simulink model "robot_uniciclo"  (R2025a)
settings: Solver=VariableStepAuto  StartTime=0.0  StopTime=10.0  RelTol=1e-3
settings Model: Creator=Bremdow  LastModifiedBy=Bremdow

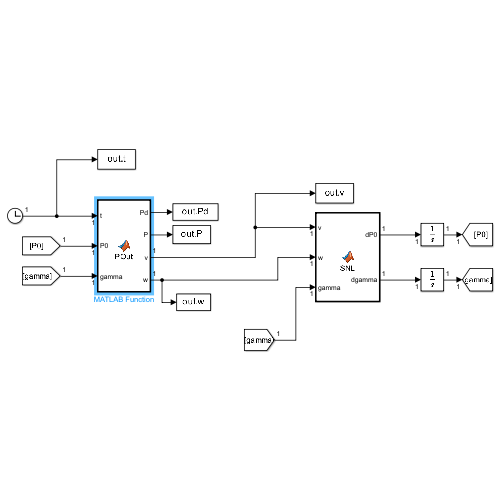
[thumbnail: Simulink's stored preview of the top-level diagram]
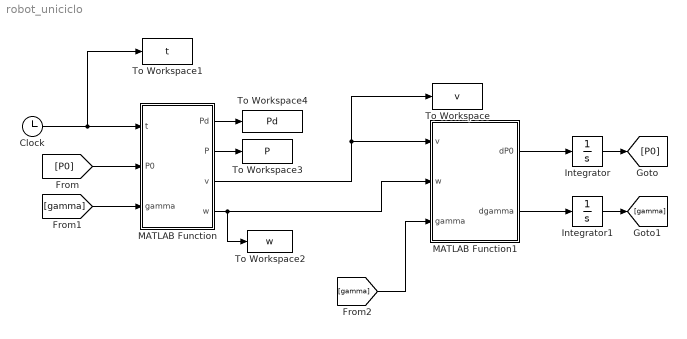
== system robot_uniciclo ==
  Clock : Clock
  Integrator : Integrator
  Integrator1 : Integrator
  MATLAB Function : MATLAB Function  TreatAsAtomicUnit=on
  MATLAB Function1 : MATLAB Function  TreatAsAtomicUnit=on
  To Workspace : ToWorkspace  VariableName=v  SampleTime=-1
  To Workspace1 : ToWorkspace  VariableName=t  SampleTime=-1
  To Workspace2 : ToWorkspace  VariableName=w  SampleTime=-1
  To Workspace3 : ToWorkspace  VariableName=P  SampleTime=-1
  To Workspace4 : ToWorkspace  VariableName=Pd  SampleTime=-1
  wires:
  Integrator/1 -> [P0]
  [gamma] -> MATLAB Function1/3(gamma)
  [gamma] -> MATLAB Function/3(gamma)
  [P0] -> MATLAB Function/2(P0)
  Clock/1 -> To Workspace1/1, MATLAB Function/1(t)
  MATLAB Function/4(w) -> MATLAB Function1/2(w), To Workspace2/1
  MATLAB Function/3(v) -> To Workspace/1, MATLAB Function1/1(v)
  MATLAB Function/2(P) -> To Workspace3/1
  MATLAB Function1/1(dP0) -> Integrator/1
  Integrator1/1 -> [gamma]
  MATLAB Function1/2(dgamma) -> Integrator1/1
  MATLAB Function/1(Pd) -> To Workspace4/1

== matlab function robot_uniciclo/MATLAB Function1 ==
  data: v input; dP0 output; w input; gamma input; dgamma output
function [dP0, dgamma] = SNL(v, w, gamma)
dP0 = [v*cos(gamma); v*sin(gamma)];
dgamma = w;

== matlab function robot_uniciclo/MATLAB Function ==
  data: t input; Pd output size=2; P0 input; gamma input; P output size=2; v output size=1; w output size=1
function [Pd, P, v, w] = POut(t, P0, gamma)
% Control PD del unicíclo tomando punto por fuera

% Parámetros del controlador
d  = 0.1;     % Distancia del punto por fuera [m]
kp = 2;       % Ganancia proporcional

% Trayectoria deseada (circunferencia)
T  = 40;
b  = 2*pi/T;

Pd  = [cos(b*t); sin(b*t)];                 % Posición deseada
dPd = [-b*sin(b*t); b*cos(b*t)];            % Velocidad deseada

% Punto por fuera
P = [P0(1) + d*cos(gamma);
     P0(2) + d*sin(gamma)];

% Error de seguimiento
e = Pd - P;

% Matriz de desacoplamiento
A = [cos(gamma), -d*sin(gamma);
     sin(gamma),  d*cos(gamma)];

% Control P con compensación
u = dPd + kp*e;
U = A \ u;      % Resolución del sistema (obtener la inversa \)

% Velocidades del unicíclo
v = U(1);       % Velocidad lineal
w = U(2);       % Velocidad angular
